simulink model "CF009A_GmOvrlStMgr"  (R2013b)
settings: Solver=FixedStepDiscrete  SolverMode=SingleTasking  StartTime=0.0  StopTime=1  FixedStep=0.002  RelTol=1e-3
values from neighbouring files (symbols this model uses):
  APASTACTV_CNT_U08 = DataDict.Constant    [CF009A_GmOvrlStMgr_DataDict.m]
  APASTCTRLAVL_CNT_U08 = DataDict.Constant    [CF009A_GmOvrlStMgr_DataDict.m]
  ARCHGLBPRM_2MILLISEC_SEC_F32 = DataDict.Constant    [CF009A_GmOvrlStMgr_DataDict.m]
  GmOvrlStMgrApaHwTqThd = DataDict.Calibration    [CF009A_GmOvrlStMgr_DataDict.m]
  GmOvrlStMgrApaHwTqTiThd = DataDict.Calibration    [CF009A_GmOvrlStMgr_DataDict.m]
  GmOvrlStMgrApaMfgEna = DataDict.Calibration    [CF009A_GmOvrlStMgr_DataDict.m]
  GmOvrlStMgrEscMfgEna = DataDict.Calibration    [CF009A_GmOvrlStMgr_DataDict.m]
  GmOvrlStMgrHaptcAmp = DataDict.Calibration    [CF009A_GmOvrlStMgr_DataDict.m]
  GmOvrlStMgrHaptcDurn = DataDict.Calibration    [CF009A_GmOvrlStMgr_DataDict.m]
  GmOvrlStMgrHaptcFrq = DataDict.Calibration    [CF009A_GmOvrlStMgr_DataDict.m]
  GmOvrlStMgrHaptcReactnTi = DataDict.Calibration    [CF009A_GmOvrlStMgr_DataDict.m]
  GmOvrlStMgrHaptcReqTiThd = DataDict.Calibration    [CF009A_GmOvrlStMgr_DataDict.m]
  GmOvrlStMgrHwAgTarLimr = DataDict.Calibration    [CF009A_GmOvrlStMgr_DataDict.m]
  GmOvrlStMgrLkaHwTqThd1 = DataDict.Calibration    [CF009A_GmOvrlStMgr_DataDict.m]
  GmOvrlStMgrLkaHwTqThd2 = DataDict.Calibration    [CF009A_GmOvrlStMgr_DataDict.m]
  GmOvrlStMgrLkaHwTqTiThd1 = DataDict.Calibration    [CF009A_GmOvrlStMgr_DataDict.m]
  GmOvrlStMgrLkaHwTqTiThd2 = DataDict.Calibration    [CF009A_GmOvrlStMgr_DataDict.m]
  GmOvrlStMgrLkaMfgEna = DataDict.Calibration    [CF009A_GmOvrlStMgr_DataDict.m]
  GmOvrlStMgrLoaMtgtnHaptcFbOffTi = DataDict.Calibration    [CF009A_GmOvrlStMgr_DataDict.m]
  GmOvrlStMgrLoaMtgtnHaptcFbOnTi = DataDict.Calibration    [CF009A_GmOvrlStMgr_DataDict.m]
  GmOvrlStMgrLoaMtgtnHaptcFbStrtOnTi = DataDict.Calibration    [CF009A_GmOvrlStMgr_DataDict.m]
  GmOvrlStMgrLoaMtgtnHaptcFbTqMax = DataDict.Calibration    [CF009A_GmOvrlStMgr_DataDict.m]
  GmOvrlStMgrLoaMtgtnHaptcFbTqMin = DataDict.Calibration    [CF009A_GmOvrlStMgr_DataDict.m]
  GmOvrlStMgrLoaMtgtnHaptcFbVehSpdMax = DataDict.Calibration    [CF009A_GmOvrlStMgr_DataDict.m]
  GmOvrlStMgrLoaMtgtnHaptcFbVehSpdMin = DataDict.Calibration    [CF009A_GmOvrlStMgr_DataDict.m]
  GmOvrlStMgrLoaMtgtnHaptcFrq = DataDict.Calibration    [CF009A_GmOvrlStMgr_DataDict.m]
  GmOvrlStMgrLoaMtgtnStrtHaptcAmp = DataDict.Calibration    [CF009A_GmOvrlStMgr_DataDict.m]
  GmOvrlStMgrLoaStIgnCntrThd = DataDict.Calibration    [CF009A_GmOvrlStMgr_DataDict.m]
  GmOvrlStMgrShiftLvrTiThd = DataDict.Calibration    [CF009A_GmOvrlStMgr_DataDict.m]
  GmOvrlStMgrStandStillThd = DataDict.Calibration    [CF009A_GmOvrlStMgr_DataDict.m]
  GmOvrlStMgrStandStillTiThd = DataDict.Calibration    [CF009A_GmOvrlStMgr_DataDict.m]
  HAPTCSTACTV_CNT_U08 = DataDict.Constant    [CF009A_GmOvrlStMgr_DataDict.m]
  HAPTCSTWAIT_CNT_U08 = DataDict.Constant    [CF009A_GmOvrlStMgr_DataDict.m]
  HWOSCNFRQMIN_HZ_F32 = DataDict.Constant    [CF009A_GmOvrlStMgr_DataDict.m]
  LKAFLTCNTRTHD_CNT_U08 = DataDict.Constant    [CF009A_GmOvrlStMgr_DataDict.m]
  LKAFLTTMRTHD_MILLISEC_U32 = DataDict.Constant    [CF009A_GmOvrlStMgr_DataDict.m]
  LKASTPRMNTFAILD_CNT_U08 = DataDict.Constant    [CF009A_GmOvrlStMgr_DataDict.m]
  MILLISECTO100MICROSECCNVN_CNT_U32 = DataDict.Constant    [CF009A_GmOvrlStMgr_DataDict.m]
  NODEBSTEP_CNT_U16 = DataDict.Constant    [CF009A_GmOvrlStMgr_DataDict.m]
undefined symbols (not defined in the file or in its folder): LoaSt1, NtcNr1, NtcSts1, NVM_RequestResultType, SysSt1
libraries: simulink x15, Fil x6, NxtrNvM x4, NxtrLim x4, NxtrAbslt x3, NxtrSign x2, FixdToFloat x1, FloatToFixd x1, LnrIntrpn x1
(part 2 of 8)

== stateflow chart CF009A_GmOvrlStMgr/GmOvrlStMgr/GmOvrlStMgrPer1/Chart ==
  state ESC [parallel]
    settings: executionOrder=1
    state Inactive
      entry:
      EscSt =ESCSTINACTV_CNT_U08 ;
    state Permanently_Failed
      entry:
      EscSt = ESCSTPRMNTFAILD_CNT_U08;
    state Active
      entry:
      EscSt = ESCSTACTV_CNT_U08;
    state Temporarily_Limited
      entry:
      EscSt = ESCSTTMPLIMD_CNT_U08;
    state Manufacturing_Disable
      entry:
      EscSt = ESCSTMFGDI_CNT_U08;
    (default) -> ESC.Inactive [order 2]
    ESC.Inactive -> ESC.Permanently_Failed [order 1] : [(EscFlt) || (LoaSt==LoaSt1.LOAST_SWBASDMTGTN)]
    ESC.Temporarily_Limited -> ESC.Inactive [order 2] : [~EscEna && (SysSt == SysSt1.SYSST_ENA)]
    ESC.Permanently_Failed -> ESC.Inactive : [((~EscEna) && (~EscFlt))&& ...
        | (LoaSt== LOASTNORM_CNT_U08)]
    ESC.Inactive -> ESC.Active [order 2] : [(EscEna) &&...
        | (VehSpdSecurMax <=GmOvrlStMgrEscVehSpdHiLim)]
    ESC.Active -> ESC.Inactive [order 2] : [(~EscEna)||...
        | (VehSpdSecurMax>GmOvrlStMgrEscVehSpdHiLim)]
    ESC.Active -> ESC.Permanently_Failed [order 1] : [EscFlt || (LoaSt==LoaSt1.LOAST_SWBASDMTGTN)]
    ESC.Temporarily_Limited -> ESC.Active [order 3] : [~EscLimdActv &&  (SysSt == SysSt1.SYSST_ENA)]
    ESC.Temporarily_Limited -> ESC.Permanently_Failed [order 1] : [(EscFlt ||...
        |  (LoaSt==LoaSt1.LOAST_SWBASDMTGTN))]
    ESC.Active -> ESC.Temporarily_Limited [order 3] : [(SysSt == SysSt1.SYSST_DI) || ...
        |  (EscLimdActv)]
    (default) -> ESC.Manufacturing_Disable [order 1] : [~EscMfgEna]
  state APA [parallel]
    settings: executionOrder=3
    state APANormal
      state TemporarilyInhibited
        entry:
        ApaSt = APASTTMPINHB_CNT_U08;
      state Available_for_Control
        entry:
        ApaSt = APASTCTRLAVL_CNT_U08;
        exit:
        HaptcSt = HAPTCSTINACTVNOTPLS_CNT_U08;
        state Not_Pulsing
          entry:
          HaptcSt = HAPTCSTINACTVNOTPLS_CNT_U08;
        state Pulsing
          state Pulse_Running
            entry:
            HaptcSt = HAPTCSTACTV_CNT_U08;
          state Waiting_After_Pulse
            entry:
            HaptcSt = HAPTCSTWAIT_CNT_U08;
          (default) -> Pulse_Running
          Pulse_Running -> Waiting_After_Pulse : [HaptcStTranActvToWaitFlg]
        state Ready_to_Pulse
          entry:
          HaptcSt = HAPTCSTINACTVRDYTOPLS_CNT_U08;
        state Pulse_Disabled
          entry:
          HaptcSt = HAPTCSTDI_CNT_U08;
        (default) -> Not_Pulsing [order 2]
        Pulsing -> Not_Pulsing : [(~VehStandStillTiExcdd) ||...
            |  (~ShiftLvrRvsTiExcdd) ||...
            |  (~ApaEna)]
        Not_Pulsing -> Ready_to_Pulse : [~HwHaptcEna]
        Ready_to_Pulse -> Not_Pulsing [order 2] : [HwHaptcEna]
        Ready_to_Pulse -> Pulsing [order 1] : [(VehStandStillTiExcdd) &&...
            |  (ShiftLvrRvsTiExcdd) &&...
            |  (ApaEna) &&...
            |  (HwHaptcEna)]
        (default) -> Pulse_Disabled [order 1] : [~GmOvrlStMgrApaHaptcEna]
      state Permanently_Failed
        entry:
        ApaSt =APASTPRMNTFAILD_CNT_U08 ;
      state Manufacturing_Disable
        entry:
        ApaSt = APASTMFGDI_CNT_U08;
      state Active
        entry:
        ApaSt =APASTACTV_CNT_U08;
      (default) -> TemporarilyInhibited [order 2]
      TemporarilyInhibited -> APA.APANormal.Permanently_Failed [order 1] : [(ApaNrcvrlFlt || ...
          | (LoaSt==LoaSt1.LOAST_SWBASDMTGTN))]
      APA.APANormal.Active -> TemporarilyInhibited [order 2] : [(SysSt == SysSt1.SYSST_DI) || ...
          |  (VehSpdSecurMax > GmOvrlStMgrApaVehSpdHiLim) ||...
          |  (ApaRcvrlFlt) ||...
          |  (HwHaptcEna) || ...
          |  (ApaIntv)]
      Available_for_Control -> TemporarilyInhibited [order 2] : [(SysSt == SysSt1.SYSST_DI) || ...
          |  (VehSpdSecurMax > GmOvrlStMgrApaVehSpdHiLim) ||...
          |  (ApaRcvrlFlt) ||...
          |  ((HwHaptcEna) && (HwHaptcEnaDurnExcdd))]
      TemporarilyInhibited -> Available_for_Control [order 2] : [(VehSpdSecurMax <= GmOvrlStMgrApaVehSpdHiLim) &&...
          |  (~ApaEna) &&...
          |  (~HwHaptcEna) &&...
          |  (~ApaRcvrlFlt)&&...
          | (SysSt == SysSt1.SYSST_ENA)]
      Available_for_Control -> APA.APANormal.Permanently_Failed [order 1] : [ApaNrcvrlFlt ||(LoaSt==LoaSt1.LOAST_SWBASDMTGTN)]
      APA.APANormal.Active -> APA.APANormal.Permanently_Failed [order 1] : [ApaNrcvrlFlt ||(LoaSt==LoaSt1.LOAST_SWBASDMTGTN)]
      Waiting_After_Pulse -> APA.APANormal.Active : [TranHaptcWaitToApaStActvFlg]
      Pulse_Disabled -> APA.APANormal.Active : [(VehStandStillTiExcdd) &&...
          |  (ShiftLvrRvsTiExcdd) &&...
          |  (ApaEna)]
      APA.APANormal.Active -> Available_for_Control [order 3] : [~ApaEna]
      (default) -> APA.APANormal.Manufacturing_Disable [order 1] : [~ApaMfgEna]
    (default) -> APANormal
  state LKA [parallel]
    settings: executionOrder=2
    state Inactive
      entry:
      LkaSt = LKASTINACTV_CNT_U08;
    state Temporarily_Limited
      entry:
      LkaSt = LKASTTMPLIMD_CNT_U08;
    state Active
      entry:
      LkaSt = LKASTACTV_CNT_U08;
    state Permanently_Failed
      entry:
      LkaSt = LKASTPRMNTFAILD_CNT_U08;
    state Manufacturing_Disable
      entry:
      LkaSt = LKASTMFGDI_CNT_U08;
    (default) -> LKA.Inactive [order 2]
    LKA.Temporarily_Limited -> LKA.Inactive [order 2] : [~LkaEna && (SysSt == SysSt1.SYSST_ENA)]
    LKA.Inactive -> LKA.Permanently_Failed [order 1] : [LkaPrmntFlt||(LoaSt==LoaSt1.LOAST_SWBASDMTGTN)]
    LKA.Inactive -> LKA.Temporarily_Limited [order 2] : [(SysSt == SysSt1.SYSST_DI) || ...
        |   ( (LkaEna) &&...
        |     ( (LkaFlt) ||...
        |       (LkaInhb) ||...
        |       (EscSt==ESCSTACTV_CNT_U08) ||...
        |       (EscSt==ESCSTTMPLIMD_CNT_U08)...
        |      )...
        |   )]
    LKA.Inactive -> LKA.Active [order 3] : [LkaEna &&...
        | (VehSpdSecurMin > GmOvrlStMgrLkaVehSpdLoLim) &&...
        | (VehSpdSecurMax < GmOvrlStMgrLkaVehSpdHiLim)]
    LKA.Active -> LKA.Inactive [order 2] : [(VehSpdSecurMin < GmOvrlStMgrLkaVehSpdLoLim) ||...
        |  (VehSpdSecurMax > GmOvrlStMgrLkaVehSpdHiLim) ||...
        |  (~LkaEna)]
    LKA.Active -> LKA.Permanently_Failed [order 1] : [LkaPrmntFlt|| (LoaSt==LoaSt1.LOAST_SWBASDMTGTN)]
    LKA.Active -> LKA.Temporarily_Limited [order 3] : [(SysSt == SysSt1.SYSST_DI) || ...
        |  ((LkaFlt) ||...
        |   (LkaInhb) ||...
        |   (LKAIntv) || ...
        |   (EscSt==ESCSTACTV_CNT_U08) || ...
        |   (EscSt==ESCSTTMPLIMD_CNT_U08)...
        |  ) ]
    LKA.Temporarily_Limited -> LKA.Permanently_Failed [order 1] : [(LkaPrmntFlt ||...
        |  (LoaSt==LoaSt1.LOAST_SWBASDMTGTN))]
    (default) -> LKA.Manufacturing_Disable [order 1] : [~LkaMfgEna]
  note: Nexteer Confidential -- Copyright 2013 Nexteer
  data: ApaSt output; VehSpdSecurMin input; VehSpdSecurMax input; ApaEna input; HwHaptcEna input; HwHaptcEnaDurnExcdd input; HaptcSt output uint8; VehStandStillTiExcdd input; ShiftLvrRvsTiExcdd input; ApaIntv input; ApaRcvrlFlt input; ApaNrcvrlFlt input; LkaSt output; LkaEna input; LkaFlt input; LkaInhb input; LkaPrmntFlt input; GmOvrlStMgrApaVehSpdHiLim parameter; GmOvrlStMgrLkaVehSpdHiLim parameter; GmOvrlStMgrLkaVehSpdLoLim parameter; GmOvrlStMgrApaHaptcEna parameter; EscSt output; EscEna input; EscFlt input; EscLimdActv input; ApaMfgEna input; LkaMfgEna input; EscMfgEna input; GmOvrlStMgrEscVehSpdHiLim parameter; LoaSt input uint8; APASTACTV_CNT_U08 parameter; APASTCTRLAVL_CNT_U08 parameter; APASTMFGDI_CNT_U08 parameter; APASTPRMNTFAILD_CNT_U08 parameter; APASTTMPINHB_CNT_U08 parameter; ESCSTACTV_CNT_U08 parameter; ESCSTINACTV_CNT_U08 parameter; ESCSTMFGDI_CNT_U08 parameter; ESCSTPRMNTFAILD_CNT_U08 parameter; ESCSTTMPLIMD_CNT_U08 parameter; HAPTCSTACTV_CNT_U08 parameter; HAPTCSTINACTVNOTPLS_CNT_U08 parameter; HAPTCSTWAIT_CNT_U08 parameter; LKASTACTV_CNT_U08 parameter; LKASTINACTV_CNT_U08 parameter; LKASTMFGDI_CNT_U08 parameter; LKASTPRMNTFAILD_CNT_U08 parameter; LKASTTMPLIMD_CNT_U08 parameter; LKAIntv input; HaptcStTranActvToWaitFlg input; TranHaptcWaitToApaStActvFlg input; HAPTCSTINACTVRDYTOPLS_CNT_U08 parameter; HAPTCSTDI_CNT_U08 parameter; SysSt input; LOASTNORM_CNT_U08 parameter

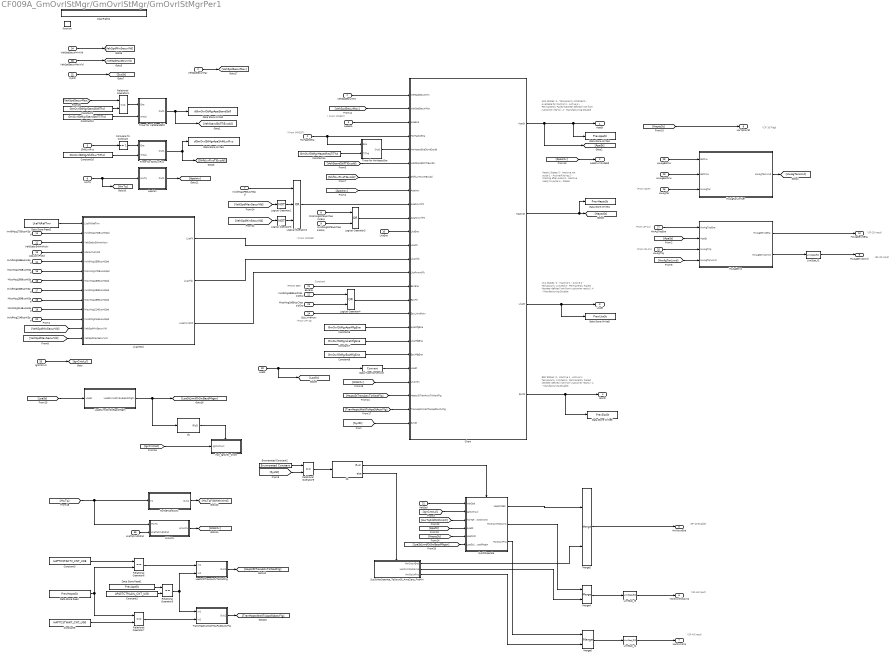
== system CF009A_GmOvrlStMgr/GmOvrlStMgr/GmOvrlStMgrPer1 ==
  note: ( From MM180)
  note: ( From MM337)
  note: ( From MM337)
  note: Constant
  note: (From SCIR)
  note: (From SF-21)
  note: (FROM SER)
  note: LKA States:
      |     0 - Inactive
      |     1 - Active
      |     2 - Temporarily Limited
      |     3 - Permanently Failed
      |
      | Nexteer defined (not from customer req'ts):
      |     4 - Manufacturing Disable
  note: APA States:
      |     0 - Temporarily Inhibited
      |     1 - Available for Control
      |     2 - Active
      |     3 - Permanently Failed
      |
      | Nexteer defined (not from customer req'ts):
      |     4 - Manufacturing Disable
  note: (SF-43 Enable)
  note: (SF-43 Input)
  note: (SF-43 Input)
  note: (CF-10 Flag)
  note: (From CF-10)
  note: ESC States:
      |     0 - Inactive
      |     1 - Active
      |     2 - Temporarily Limited
      |     3 - Permanently Failed
      |
      | Nexteer defined (not from customer req'ts):
      |     4 - Manufacturing Disable
  note: Haptic States
      |     0 - Inactive not pulse
      |     1 - Active/Pulsing
      |     2 - Waiting after pulse
      |     3 - Inactive ready to pulse
      |     4 - Diable
  note: (SF-20 Input)
  note: (SF-20 Input)
  note: (From SF-21)
  VehSpdSecurMin : Inport  RequirementInfo={} %GIDa_b0d3c35c_4503_4005_8ea2_9f2212553c6a
  VehSpdSecurMax : Inport  RequirementInfo={} %GIDa_e53e6896_dd80_42dc_965a_fcb79ee9124b  Port=2
  ApaEna : Inport  RequirementInfo={} %GIDa_8d1b5d03_8c5e_4c5e_91f3_bdd695e85069  Port=3
  HwHaptcEna : Inport  RequirementInfo={} %GIDa_06485b27_ab40_4ad3_bd14_ad4c2f62a393  Port=4
  ShiftLvrRvs : Inport  RequirementInfo={} %GIDa_dbbb7a9a_4381_48ec_960c_58daf9f19689  Port=5
  HwTq : Inport  RequirementInfo={} %GIDa_1ba3b84f_cb31_41a6_8598_2ca61152b6d2  Port=6
  InvldMsg1F5BusHiSpd : Inport  RequirementInfo={} %GIDa_f9b8db8c_5ec9_4279_8101_3b3cb8e96ee5  Port=7
  MissMsg337BusChassisExp : Inport  RequirementInfo={} %GIDa_2a54828a_623d_4a68_a97f_ee6c81b0f13e  Port=8
  InvldMsg337BusChassisExp : Inport  RequirementInfo={} %GIDa_a49582db_91ce_41e4_8ea7_fdb3beb7f641  Port=9
  LkaEna : Inport  RequirementInfo={} %GIDa_c67f821d_a534_4859_991f_be754908d78a  Port=10
  InvldMsg17DBusHiSpd : Inport  RequirementInfo={} %GIDa_c076c772_eeab_449c_b484_472e0cc8ed94  Port=11
  VehStabyEnhmtActv : Inport  RequirementInfo={} %GIDa_d5abf950_7af4_40d5_9676_0be52ecf66dc  Port=12
  AbsActvProtd : Inport  RequirementInfo={} %GIDa_04825455_bd19_4a90_9118_99efddee4468  Port=13
  InvldMsg1E9BusHiSpd : Inport  RequirementInfo={} %GIDa_ac4e6f02_8e0b_4fad_9ad8_288bf6f696c2  Port=14
  MissMsg17DBusHiSpd : Inport  RequirementInfo={} %GIDa_fcbc91b2_5e8e_4fde_b293_feb4eb68ea1d  Port=15
  MissMsg180BusHiSpd : Inport  RequirementInfo={} %GIDa_5a4e98da_8e0e_4ded_8f2b_0b345abaefca  Port=16
  InvldMsg180BusHiSpd : Inport  RequirementInfo={} %GIDa_c8d0ce3f_644b_4f0b_b33b_1e2f6d27c9df  Port=17
  MissMsg1E9BusHiSpd : Inport  RequirementInfo={} %GIDa_6ee56723_44b7_42b6_81ab_70915cbf1039  Port=18
  MissMsg214BusHiSpd : Inport  RequirementInfo={} %GIDa_9b7d257f_e0dc_4c9e_80ad_4a379171a5c2  Port=19
  InvldMsg214BusHiSpd : Inport  RequirementInfo={} %GIDa_ac526c57_18d5_4464_a148_218d3bfa9251  Port=20
  EscEna : Inport  RequirementInfo={} %GIDa_b7127805_3263_4184_831a_fc6c9b2cc01a  Port=21
  InvldMsg180BusChassisExp : Inport  RequirementInfo={} %GIDa_9ef29787_08e6_4663_a122_36a87bb12d59  Port=22
  MissMsg180BusChassisExp : Inport  RequirementInfo={} %GIDa_58661bb7_935e_4aa5_b2cb_a8077cff621a  Port=23
  EscLimdActv : Inport  RequirementInfo={} %GIDa_b1f90e60_6bab_4611_8ad9_e41738359040  Port=24
  HwAgTraj : Inport  RequirementInfo={} %GIDa_d5ec0ae6_f9e7_41b2_bf71_b480815ec2e8  Port=25
  HwAgTar : Inport  RequirementInfo={} %GIDa_6d588383_a210_4589_8f75_f9a00bf487c4  Port=26
  HwAgTrajEna : Inport  RequirementInfo={} %GIDa_30a153ec_8bbd_4ae8_86d5_91622ecf057d  Port=27
  HwAgEotCw : Inport  RequirementInfo={} %GIDa_a50a5d22_edbb_46ee_a5b7_bf143e2be1e6  Port=28
  HwAgEotCcw : Inport  RequirementInfo={} %GIDa_e08702f0_b186_40e1_9d5d_bab753fad415  Port=29
  LoaSt : Inport  RequirementInfo={} %GIDa_6f65a69f_1af1_4842_b860_3f517f73d3e8  Port=30  OutDataTypeStr=Enum: LoaSt1
  VehSpd : Inport  RequirementInfo={} %GIDa_198a1be4_59f5_4e8c_9975_df192cdf1251  Port=31
  SysSt : Inport  RequirementInfo={} %GIDa_5d1f0e27_a7b9_4b52_8773_b774a1daf0f1  Port=32
  IgnCntrLcl : Inport  RequirementInfo={} %GIDa_e0ba004e_4503_44da_8652_b13ad7bc9694  Port=33
  VehSpdSecurMinVld : Inport  RequirementInfo={} %GIDa_8aa24ca1_68b2_4a9c_89a4_0495831d4359  Port=34
  VehSpdSecurMaxVld : Inport  RequirementInfo={} %GIDa_dc311978_557e_4d2a_9a37_0f77a83cb914  Port=35
  "LkaTqCmdCdnd " : Inport  RequirementInfo={} %GIDa_6a679366_d481_4ed4_897f_c24ea9a03044  Port=36
  function : TriggerPort  TriggerType=function-call  PortDimensions=1
  ApaIntv : Subsystem
  Chart : Stateflow chart  RequirementInfo="{}  %GIDa_82f8cf8a_e966_40c9_996b_fc039507f794"  TreatAsAtomicUnit=on
  Compare To Constant : simulink/Logic and Bit Operations/Compare To Constant  relop===  const=1  OutDataTypeStr=boolean
  Constant1 : Constant  RequirementInfo={} %GIDa_7552fffd_837c_418f_a626_cb54a4ee4ecb  Value=GmOvrlStMgrStandStillThd
  Constant12 : Constant  RequirementInfo={} %GIDa_e0385d72_a04c_4c7f_8712_c1743adc4cad  Value=GmOvrlStMgrStandStillTiThd
  Constant14 : Constant  RequirementInfo={} %GIDa_4c34fc80_0be8_4916_b589_f77a913bde0d  Value=GmOvrlStMgrHaptcReqTiThd
  Constant16 : Constant  RequirementInfo={} %GIDa_414bbb4b_0344_45a0_913d_45c0053809cf  Value=GmOvrlStMgrShiftLvrTiThd
  Constant2 : Constant  Value=APASTCTRLAVL_CNT_U08
  Constant3 : Constant  Value=HAPTCSTACTV_CNT_U08
  Constant5 : Constant  Value=HAPTCSTWAIT_CNT_U08
  Constant6 : Constant  RequirementInfo={} %GIDa_6b44c89b_d793_4fde_b6dc_5afdec075d44  Value=GmOvrlStMgrApaMfgEna
  Constant7 : Constant  RequirementInfo={} %GIDa_f42bd636_c9a1_4d24_9506_dba1aeb30581  Value=GmOvrlStMgrLkaMfgEna
  Constant8 : Constant  RequirementInfo={} %GIDa_d43e135b_4699_428a_b5cf_b127f48922b5  Value=GmOvrlStMgrEscMfgEna
  CopyRight2 : Subsystem  Description=|  mask(Copyright Information){none=on}
      | Copyright info block.                                               
      |                                                                     
      | Place copyright information at the top of every subsystem in design.
      mask prompts: none "No parameters"
      mask help: Place copyright information at the top of every subsystem in design.
      mask Display:
      | NxtrConf = 'Nexteer Confidential';
      | 
      | sys = bdroot; %handle for the current model ("system")
      | first = get_param(sys,'Created');
      | first = first(end-3:end);  %year is last four digits
      | 
      | last = get_param(sys,'LastModifiedDate');
      | if isempty(last)
      |     last = datestr(now,'yyyy');
      | else
      |     last = last(end-3:end);
      | end
      | 
      | if strcmp(first,last)
      |     fprintf('%s -- Copyright %s Nexteer',NxtrConf,first)
      | else
      |     fprintf('%s -- %s%s- %s Nexteer',NxtrConf,char(169),first,last)
      | end
  Data Store Read : DataStoreRead  DataStoreName=PrevHaptcSt
  Data Store Read1 : DataStoreRead  DataStoreName=PrevApaSt
  Data Store Read2 : DataStoreRead  DataStoreName=LkaFltRefTmr
  Data Store Write1 : DataStoreWrite  DataStoreName=dGmOvrlStMgrApaShiftLvrRvs
  Data Store Write2 : DataStoreWrite  DataStoreName=dGmOvrlStMgrApaStandStill
  Data Store Write3 : DataStoreWrite  DataStoreName=PrevApaSt
  Data Store Write4 : DataStoreWrite  DataStoreName=PrevHaptcSt
  Data Store Write5 : DataStoreWrite  DataStoreName=PrevLkaSt
  Data Store Write6 : DataStoreWrite  DataStoreName=PrevEscSt
  Data Type Conversion : DataTypeConversion
  Enumerated Constant2 : simulink/Sources/Enumerated Constant  OutDataTypeStr=Enum: SysSt1  Value=SysSt1.SYSST_ENA  SampleTime=inf
  HaptcStTransActvToWaitFlg : Subsystem
  HwAgServo : Subsystem  RequirementInfo={} %GIDa_aaea10c3_5552_4f84_b64c_db5f293fc08c
  HwAgTarLimiter : Subsystem  RequirementInfo={} %GIDa_1c9b0e23_9620_4264_8618_d0192b732e95
  HwTqFildIntlChk : Subsystem
  If1 : If  IfExpression=u1  ShowElse=off
  If4 : If  IfExpression=u1
  Inct_IgnCntr_Once : Subsystem
  LKAIntv : Subsystem
  LimStat_f1 : NxtrLim/LimStat_f32  LoLim=HWAGSERVOCMDMIN_HWDEG_F32  HiLim=HWAGSERVOCMDMAX_HWDEG_F32
      settings: AttributesFormatString=|
      | Low Limit: %<LoLim>
      | High Limit:%<HiLim>
  LimStat_f3 : NxtrLim/LimStat_f32  LoLim=HWOSCNMOTAMPMIN_MOTNWTMTR_F32  HiLim=HWOSCNMOTAMPMAX_MOTNWTMTR_F32
      settings: AttributesFormatString=|
      | Low Limit: %<LoLim>
      | High Limit:%<HiLim>
  LimStat_f4 : NxtrLim/LimStat_f32  LoLim=HWOSCNFRQMIN_HZ_F32  HiLim=HWOSCNFRQMAX_HZ_F32
      settings: AttributesFormatString=|
      | Low Limit: %<LoLim>
      | High Limit:%<HiLim>
  LkaCheck : Subsystem
  LoaStLimdOrSwBasdMtgtn : Subsystem
  Logical Operator1 : Logic  Operator=NOT  AllPortsSameDT=off  OutDataTypeStr=boolean
  Logical Operator2 : Logic  Operator=OR  Inputs=3  AllPortsSameDT=off  OutDataTypeStr=boolean
  Logical Operator3 : Logic  Operator=OR  AllPortsSameDT=off  OutDataTypeStr=boolean
  Logical Operator4 : Logic  Operator=OR  AllPortsSameDT=off  OutDataTypeStr=boolean
  Logical Operator5 : Logic  Operator=NOT  AllPortsSameDT=off  OutDataTypeStr=boolean
  Merge4 : Merge
  Merge5 : Merge
  Merge6 : Merge
  Relational Operator3 : RelationalOperator  Operator=<=  OutDataTypeStr=boolean
  Relational Operator{5..7,9} (4 alike) : RelationalOperator  Operator===  OutDataTypeStr=boolean
  SysStNotOperate_TqOscnDi_AmpZero_FrqMin : Subsystem
  SysStOperate : Subsystem  TreatAsAtomicUnit=on
  Timer for HwHaptcEna : Subsystem
  Timer for ShiftLvrRvs : Subsystem
  Timer for VehStandStill : Subsystem
  TransHaptcsWaitToAPAStActvFlg : Subsystem
  ApaSt : Outport  RequirementInfo={} %GIDa_75635ebd_fcf5_4cad_9536_b406ee611602
  ApaDrvrIntvDetd : Outport  RequirementInfo={} %GIDa_1797abc3_35b6_41e8_9538_2064f4102f87  Port=2
  LkaSt : Outport  RequirementInfo={} %GIDa_686c82ef_a42d_4546_a1da_a62cef7fe954  Port=3
  EscSt : Outport  RequirementInfo={} %GIDa_ad72c3fe_3139_49da_a979_17fad9a56d26  Port=4
  HwOscnEna : Outport  RequirementInfo={} %GIDa_d848a758_683b_4a9d_a345_2c9338079af2  Port=5
  HwOscnMotAmp : Outport  RequirementInfo={} %GIDa_159c2416_70a4_4698_a3a2_bfc8caad832f  Port=6
  HwOscnFrq : Outport  RequirementInfo={} %GIDa_bf0dab85_578c_4235_861d_cc8928b85320  Port=7
  HwTqOscSt : Outport  RequirementInfo={} %GIDa_f57d728d_5e71_4f6a_bae2_eb0c6758b489  Port=8
  HwAgServoCmd : Outport  RequirementInfo={} %GIDa_a0e1e034_04e0_4255_bc05_d7a545e9e511  Port=9
  HwAgServoEna : Outport  RequirementInfo={} %GIDa_e4571625_3f2f_4611_bb8a_43a258de8b52  Port=10
  wires:
  EscLimdActv/1 -> Chart/17(EscLimdActv)
  HwAgTraj/1 -> HwAgServo/3(HwAgTraj)
  HwAgTar/1 -> HwAgTarLimiter/3(HwAgTar)
  Chart/1(ApaSt) -> ApaSt/1, Data Store Write3/1, [ApaSt]
  EscEna/1 -> Chart/15(EscEna)
  HwAgEotCcw/1 -> HwAgTarLimiter/2(EotCcw)
  HwHaptcEna/1 -> Timer for HwHaptcEna/1(Ena), Chart/4(HwHaptcEna)
  [HaptcSt] -> HwTqOscSt/1
  Logical Operator4/1 -> Chart/16(EscFlt)
  HwAgTarLimiter/1(HwAgTarLimd) -> [HwAgTarLimd]
  ApaEna/1 -> Chart/3(ApaEna)
  Chart/4(EscSt) -> EscSt/1, Data Store Write6/1
  Chart/3(LkaSt) -> LkaSt/1, Data Store Write5/1
  HwAgServo/1(HwAgServoEna) -> HwAgServoEna/1
  Logical Operator2/1 -> Chart/9(ApaRcvrlFlt)
  HwAgTrajEna/1 -> HwAgServo/1(HwAgTrajEna)
  HwAgEotCw/1 -> HwAgTarLimiter/1(EotCw)
  Timer for HwHaptcEna/1(Out1) -> Chart/5(HwHaptcEnaDurnExcdd)
  Chart/2(HaptcSt) -> Data Store Write4/1, [HaptcSt]
  HwAgServo/2(HwAgServoCmd) -> LimStat_f1/1
  [ApaIntv] -> ApaDrvrIntvDetd/1
  [HwAgTarLimd] -> HwAgServo/4(HwAgTarLimd)
  Logical Operator3/1 -> Chart/10(ApaNrcvrlFlt)
  LoaSt/1 -> Data Type Conversion/1, [LoaSt]
  Constant14/1 -> Timer for HwHaptcEna/2(TiThd)
  ApaIntv/1(Out1) -> [ApaIntv]
  [ApaIntv] -> Chart/8(ApaIntv)
  Timer for VehStandStill/1(Out1) -> [VehStandStillTiExcdd], Data Store Write2/1
  [VehStandStillTiExcdd] -> Chart/6(VehStandStillTiExcdd)
  Timer for ShiftLvrRvs/1(Out1) -> [ShiftLvrRvsTiExcdd], Data Store Write1/1
  ShiftLvrRvs/1 -> Compare To Constant/1
  [ShiftLvrRvsTiExcdd] -> Chart/7(ShiftLvrRvsTiExcdd)
  [VehSpdSecurMax] -> Chart/2(VehSpdSecurMax)
  [ApaSt] -> HwAgServo/2(ApaSt)
  LkaEna/1 -> Chart/11(LkaEna)
  Constant12/1 -> Timer for VehStandStill/2(TiThd)
  Constant1/1 -> Relational Operator3/2
  Relational Operator3/1 -> Timer for VehStandStill/1(Ena)
  Constant16/1 -> Timer for ShiftLvrRvs/2(TiThd)
  Compare To Constant/1 -> Timer for ShiftLvrRvs/1(Ena)
  InvldMsg1F5BusHiSpd/1 -> Logical Operator2/1
  InvldMsg337BusChassisExp/1 -> Logical Operator3/2
  MissMsg337BusChassisExp/1 -> Logical Operator3/1
  InvldMsg180BusChassisExp/1 -> Logical Operator4/1
  MissMsg180BusChassisExp/1 -> Logical Operator4/2
  HwTq/1 -> [HwTq], ApaIntv/1(HwTq)
  Data Type Conversion/1 -> Chart/21(LoaSt)
  LimStat_f3/1 -> HwOscnMotAmp/1
  LimStat_f4/1 -> HwOscnFrq/1
  HwTqFildIntlChk/1(Out1) -> [HwTqFildWithinIntl]
  LKAIntv/1(LKAIntv) -> [LKAIntv]
  [LKAIntv] -> Chart/22(LKAIntv)
  LimStat_f1/1 -> HwAgServoCmd/1
  HaptcStTransActvToWaitFlg/1(Out1) -> [HaptcStTranActvToWaitFlg]
  TransHaptcsWaitToAPAStActvFlg/1(Out1) -> [TranHaptcWaitToApaStActvFlg]
  [HaptcStTranActvToWaitFlg] -> Chart/23(HaptcStTranActvToWaitFlg)
  [TranHaptcWaitToApaStActvFlg] -> Chart/24(TranHaptcWaitToApaStActvFlg)
  Data Store Read1/1 -> Relational Operator5/1
  Constant2/1 -> Relational Operator5/2
  Relational Operator5/1 -> TransHaptcsWaitToAPAStActvFlg/1(In1), HaptcStTransActvToWaitFlg/2(In2)
  Constant3/1 -> Relational Operator6/1
  Data Store Read/1 -> Relational Operator7/1, Relational Operator6/2
  Constant5/1 -> Relational Operator7/2
  Relational Operator7/1 -> TransHaptcsWaitToAPAStActvFlg/2(In2)
  Relational Operator6/1 -> HaptcStTransActvToWaitFlg/1(In1)
  If4/1 -> SysStOperate/Action
  If4/2 -> SysStNotOperate_TqOscnDi_AmpZero_FrqMin/Action
  Relational Operator9/1 -> If4/1
  Enumerated Constant2/1 -> Relational Operator9/1
  SysStOperate/2(HwOscnMotAmp) -> Merge4/1
  SysStOperate/1(HaptcFbEn) -> Merge5/1
  SysStOperate/3(HwOscnFrq) -> Merge6/1
  SysStNotOperate_TqOscnDi_AmpZero_FrqMin/1(HwOscnEna) -> Merge5/2
  SysStNotOperate_TqOscnDi_AmpZero_FrqMin/3(HwOscnFrq) -> Merge6/2
  SysStNotOperate_TqOscnDi_AmpZero_FrqMin/2(HwOscnMotAmp) -> Merge4/2
  Merge5/1 -> HwOscnEna/1
  Merge6/1 -> LimStat_f4/1
  Merge4/1 -> LimStat_f3/1
  VehSpd/1 -> SysStOperate/1(VehSpd)
  [ApaSt] -> SysStOperate/4(ApaSt)
  [HaptcSt] -> SysStOperate/5(HaptcSt)
  [HwTqFildWithinIntl] -> SysStOperate/3(HwTqFildWithinIntl)
  Constant6/1 -> Chart/18(ApaMfgEna)
  Constant7/1 -> Chart/19(LkaMfgEna)
  Constant8/1 -> Chart/20(EscMfgEna)
  [IgnCntrLcl] -> SysStOperate/2(IgnCntrLcl)
  If1/1 -> Inct_IgnCntr_Once/Action
  LoaStLimdOrSwBasdMtgtn/1(LoaStLimdOrSwBasdMtgtn) -> [LoaStLimdOrSwBasdMtgtn], If1/1
  [IgnCntrLcl] -> Inct_IgnCntr_Once/1(IgnCntrLcl)
  [LoaSt] -> LoaStLimdOrSwBasdMtgtn/1(LoaSt)
  IgnCntrLcl/1 -> [IgnCntrLcl]
  [LoaStLimdOrSwBasdMtgtn] -> SysStOperate/6(LoaStLimdOrSwBasdMtgtn)
  [VehSpdSecurMax] -> Relational Operator3/1
  VehSpdSecurMin/1 -> Chart/1(VehSpdSecurMin)
  [VehSpdMaxSecurVld] -> Logical Operator1/1
  [VehSpdMinSecurVld] -> Logical Operator5/1
  LkaCheck/1(LkaFlt) -> Chart/12(LkaFlt)
  InvldMsg17DBusHiSpd/1 -> LkaCheck/2(InvldMsg17DBusHiSpd)
  VehStabyEnhmtActv/1 -> LkaCheck/3(VehStabyEnhmtActv)
  AbsActvProtd/1 -> LkaCheck/4(AbsActvProtd)
  InvldMsg1E9BusHiSpd/1 -> LkaCheck/5(InvldMsg1E9BusHiSpd)
  MissMsg17DBusHiSpd/1 -> LkaCheck/6(MissMsg17DBusHiSpd)
  MissMsg180BusHiSpd/1 -> LkaCheck/7(MissMsg180BusHiSpd)
  InvldMsg180BusHiSpd/1 -> LkaCheck/8(InvldMsg180BusHiSpd)
  MissMsg1E9BusHiSpd/1 -> LkaCheck/9(MissMsg1E9BusHiSpd)
  MissMsg214BusHiSpd/1 -> LkaCheck/10(MissMsg214BusHiSpd)
  InvldMsg214BusHiSpd/1 -> LkaCheck/11(InvldMsg214BusHiSpd)
  LkaCheck/2(LkaInhb) -> Chart/13(LkaInhb)
  LkaCheck/3(LkaPrmntFlt) -> Chart/14(LkaPrmntFlt)
  [VehSpdMaxSecurVld] -> LkaCheck/13(VehSpdMaxSecurVld)
  [VehSpdMinSecurVld] -> LkaCheck/12(VehSpdMinSecurVld)
  SysSt/1 -> [SysSt]
  [SysSt] -> Relational Operator9/2
  [SysSt] -> Chart/25(SysSt)
  VehSpdSecurMinVld/1 -> [VehSpdMinSecurVld]
  VehSpdSecurMaxVld/1 -> [VehSpdMaxSecurVld]
  Logical Operator1/1 -> Logical Operator2/2
  Logical Operator5/1 -> Logical Operator2/3
  VehSpdSecurMax/1 -> [VehSpdSecurMax]
  Data Store Read2/1 -> LkaCheck/1(LkaFltRefTmr)
  [HwTq] -> LKAIntv/1(HwTq), HwTqFildIntlChk/1(In1)
  "LkaTqCmdCdnd "/1 -> LKAIntv/2(LkaTqCmdCdnd)

== system CF009A_GmOvrlStMgr/GmOvrlStMgr/SetGmLoaIgnCntr ==
  GmLoaIgnCntr : Inport  RequirementInfo={} %GIDa_f6a28945_b2be_4817_8103_f6fab52ae2d6
  function : TriggerPort  TriggerType=function-call
  Constant1 : Constant  Value=true  OutDataTypeStr=boolean
      settings: AttributesFormatString=%<OutDataTypeStr>
  CopyRight2 : Subsystem  Description=|  mask(Copyright Information){none=on}
      | Copyright info block.                                               
      |                                                                     
      | Place copyright information at the top of every subsystem in design.
      mask prompts: none "No parameters"
      mask help: Place copyright information at the top of every subsystem in design.
      mask Display:
      | NxtrConf = 'Nexteer Confidential';
      | 
      | sys = bdroot; %handle for the current model ("system")
      | first = get_param(sys,'Created');
      | if(isempty(first))
      |     first = datestr(now,'yyyy');
      | else
      |     first = first(end-3:end);  %year is last four digits
      | end
      | 
      | last = get_param(sys,'LastModifiedDate');
      | if isempty(last)
      |     last = datestr(now,'yyyy');
      | else
      |     last = last(end-3:end);
      | end
      | 
      | if strcmp(first,last)
      |     fprintf('%s -- Copyright %s Nexteer',NxtrConf,first)
      | else
      |     fprintf('%s -- %s%s- %s Nexteer',NxtrConf,char(169),first,last)
      | end
  Data Store Write8 : DataStoreWrite  DataStoreName=GmLoaIgnCntr
  GmLoaIgnCntr_Set Ram Block Status : NxtrNvM/Set Ram Block Status  FuncName=Set Ram Block Status  NvMBlockName=GmLoaIgnCntr  VoidFuncRtn=on  BlockChanged_DSN=NvMSRBS_BlockChanged  Return_DSN=NvMSRBS_Return1
      settings: AttributesFormatString=%<FuncName>
  wires:
  GmLoaIgnCntr/1 -> Data Store Write8/1
  Constant1/1 -> GmLoaIgnCntr_Set Ram Block Status/1

== system CF009A_GmOvrlStMgr/call_GetGmLoaIgnCntr/CopyRight1 ==

== system CF009A_GmOvrlStMgr/call_GmOvrlStMgrInit1/CopyRight2 ==

== system CF009A_GmOvrlStMgr/call_GmOvrlStMgrPer1/CopyRight2 ==

== system CF009A_GmOvrlStMgr/call_SetGmLoaIgnCntr/CopyRight1 ==

== system CF009A_GmOvrlStMgr/GmOvrlStMgr/GetGmLoaIgnCntr/CopyRight2 ==

== system CF009A_GmOvrlStMgr/GmOvrlStMgr/GmOvrlStMgrInit1/CopyRight2 ==

== system CF009A_GmOvrlStMgr/GmOvrlStMgr/GmOvrlStMgrInit1/GetRefTmr100MicroSec32bit ==
  note: Created Aug 18, 2015
      | Modified Oct 21, 2015
      | Modified Oct 30, 2015
      | Kevin Derry
  note: GetRefTmr100MicroSec32bit
  note: Wrap-to-zero
  note: counts
  note: microseconds
  note: seconds
  note: 1 count = 100 uSec
  CopyRight2 : Subsystem  Description=|  mask(Copyright Information){none=on}
      | Copyright info block.                                               
      |                                                                     
      | Place copyright information at the top of every subsystem in design.
      mask prompts: none "No parameters"
      mask help: Place copyright information at the top of every subsystem in design.
      mask Display:
      | NxtrConf = 'Nexteer Confidential';
      | 
      | sys = bdroot; %handle for the current model ("system")
      | first = get_param(sys,'Created');
      | if(isempty(first))
      |     first = datestr(now,'yyyy');
      | else
      |     first = first(end-3:end);  %year is last four digits
      | end
      | 
      | last = get_param(sys,'LastModifiedDate');
      | if isempty(last)
      |     last = datestr(now,'yyyy');
      | else
      |     last = last(end-3:end);
      | end
      | 
      | if strcmp(first,last)
      |     fprintf('%s -- Copyright %s Nexteer',NxtrConf,first)
      | else
      |     fprintf('%s -- %s%s- %s Nexteer',NxtrConf,char(169),first,last)
      | end
  Count per uSec : Constant  Value=0.01
  Data Store Read1 : DataStoreRead  DataStoreName=SimnTi
  Data Type Conversion1 : DataTypeConversion  OutDataTypeStr=uint32
  Divide1 : Product  Inputs=**
  Divide2 : Product  Inputs=*/
  Max Counts : Constant  Value=2^32-1
  Product1 : Product
  Product2 : Product
  Rounding : Rounding
  Subtract1 : Sum  Inputs=+-
  uSec per Sec : Constant  Value=1000000
  RefTmr : Outport
  wires:
  Data Store Read1/1 -> Product1/1
  Data Type Conversion1/1 -> RefTmr/1
  uSec per Sec/1 -> Product1/2
  Count per uSec/1 -> Divide1/2
  Product1/1 -> Divide1/1
  Divide1/1 -> Subtract1/1, Divide2/1
  Max Counts/1 -> Product2/2, Divide2/2
  Divide2/1 -> Rounding/1
  Rounding/1 -> Product2/1
  Subtract1/1 -> Data Type Conversion1/1
  Product2/1 -> Subtract1/2

== system CF009A_GmOvrlStMgr/GmOvrlStMgr/GmOvrlStMgrInit1/NTC_Fault1_Set_Faild ==
  NtcNr : Inport
  NtcStInfo : Inport  Port=2
  NtcSts : Inport  Port=3
  DebStep : Inport  Port=4
  CallDiagMgr : ActionPort  ActionType=then
  SetNtcSts : Subsystem  RequirementInfo={} %GIDa_d459548b_e0d4_4661_8326_6b6064fa956f  TreatAsAtomicUnit=on
      settings: RTWSystemCode=Inline
  wires:
  NtcStInfo/1 -> SetNtcSts/2(NtcStInfo)
  DebStep/1 -> SetNtcSts/4(DebStep)
  NtcSts/1 -> SetNtcSts/3(NtcSts)
  NtcNr/1 -> SetNtcSts/1(NtcNr)  "NtcNr"

== system CF009A_GmOvrlStMgr/GmOvrlStMgr/GmOvrlStMgrInit1/NTC_Fault1_Set_Passd ==
  NtcNr : Inport
  NtcStInfo : Inport  Port=2
  NtcSts : Inport  Port=3
  DebStep : Inport  Port=4
  CallDiagMgr : ActionPort  ActionType=else
  SetNtcSts : Subsystem  RequirementInfo={} %GIDa_e624de36_990e_40b1_800e_f81e88e68b40  TreatAsAtomicUnit=on
      settings: RTWSystemCode=Inline
  wires:
  NtcNr/1 -> SetNtcSts/1(NtcNr)  "NtcNr"
  NtcSts/1 -> SetNtcSts/3(NtcSts)
  DebStep/1 -> SetNtcSts/4(DebStep)
  NtcStInfo/1 -> SetNtcSts/2(NtcStInfo)

== system CF009A_GmOvrlStMgr/GmOvrlStMgr/GmOvrlStMgrInit1/NVM_NOK ==
  note: In the event of NVM failure
      | zero out the shadow ram image
  Action Port : ActionPort  ActionType=then
  Constant1 : Constant  Value=0  OutDataTypeStr=uint16
      settings: AttributesFormatString=%<OutDataTypeStr>
  CopyRight2 : Subsystem  Description=|  mask(Copyright Information){none=on}
      | Copyright info block.                                               
      |                                                                     
      | Place copyright information at the top of every subsystem in design.
      mask prompts: none "No parameters"
      mask help: Place copyright information at the top of every subsystem in design.
      mask Display:
      | NxtrConf = 'Nexteer Confidential';
      | 
      | sys = bdroot; %handle for the current model ("system")
      | first = get_param(sys,'Created');
      | if(isempty(first))
      |     first = datestr(now,'yyyy');
      | else
      |     first = first(end-3:end);  %year is last four digits
      | end
      | 
      | last = get_param(sys,'LastModifiedDate');
      | if isempty(last)
      |     last = datestr(now,'yyyy');
      | else
      |     last = last(end-3:end);
      | end
      | 
      | if strcmp(first,last)
      |     fprintf('%s -- Copyright %s Nexteer',NxtrConf,first)
      | else
      |     fprintf('%s -- %s%s- %s Nexteer',NxtrConf,char(169),first,last)
      | end
  Data Store Write8 : DataStoreWrite  DataStoreName=GmLoaIgnCntr
  wires:
  Constant1/1 -> Data Store Write8/1

== system CF009A_GmOvrlStMgr/GmOvrlStMgr/GmOvrlStMgrInit1/NVM_Ok ==
  Action Port : ActionPort  ActionType=else
  Constant1 : Constant  Value=0  OutDataTypeStr=Inherit: Inherit via back propagation
  CopyRight2 : Subsystem  Description=|  mask(Copyright Information){none=on}
      | Copyright info block.                                               
      |                                                                     
      | Place copyright information at the top of every subsystem in design.
      mask prompts: none "No parameters"
      mask help: Place copyright information at the top of every subsystem in design.
      mask Display:
      | NxtrConf = 'Nexteer Confidential';
      | 
      | sys = bdroot; %handle for the current model ("system")
      | first = get_param(sys,'Created');
      | if(isempty(first))
      |     first = datestr(now,'yyyy');
      | else
      |     first = first(end-3:end);  %year is last four digits
      | end
      | 
      | last = get_param(sys,'LastModifiedDate');
      | if isempty(last)
      |     last = datestr(now,'yyyy');
      | else
      |     last = last(end-3:end);
      | end
      | 
      | if strcmp(first,last)
      |     fprintf('%s -- Copyright %s Nexteer',NxtrConf,first)
      | else
      |     fprintf('%s -- %s%s- %s Nexteer',NxtrConf,char(169),first,last)
      | end
  Terminator : Terminator
  wires:
  Constant1/1 -> Terminator/1

== system CF009A_GmOvrlStMgr/GmOvrlStMgr/GmOvrlStMgrInit1/Saturate ==
  In1 : Inport
  Action Port : ActionPort  ActionType=else
  Out1 : Outport
  wires:
  In1/1 -> Out1/1

== system CF009A_GmOvrlStMgr/GmOvrlStMgr/GmOvrlStMgrInit1/StepDown ==
  Acc : Inport
  Action Port : ActionPort  ActionType=then
  Constant1 : Constant  OutDataTypeStr=Inherit: Inherit via back propagation
  Constant8 : Constant  Value=true  OutDataTypeStr=boolean
      settings: AttributesFormatString=%<OutDataTypeStr>
  GmLoaIgnCntr_Set Ram Block Status : NxtrNvM/Set Ram Block Status  FuncName=Set Ram Block Status  NvMBlockName=GmLoaIgnCntr  VoidFuncRtn=on  BlockChanged_DSN=NvMSRBS_BlockChanged  Return_DSN=NvMSRBS_Return2
      settings: AttributesFormatString=%<FuncName>
  subtract : Sum  Inputs=+-
  NewAccum : Outport
  wires:
  subtract/1 -> NewAccum/1
  Constant1/1 -> subtract/2
  Acc/1 -> subtract/1
  Constant8/1 -> GmLoaIgnCntr_Set Ram Block Status/1

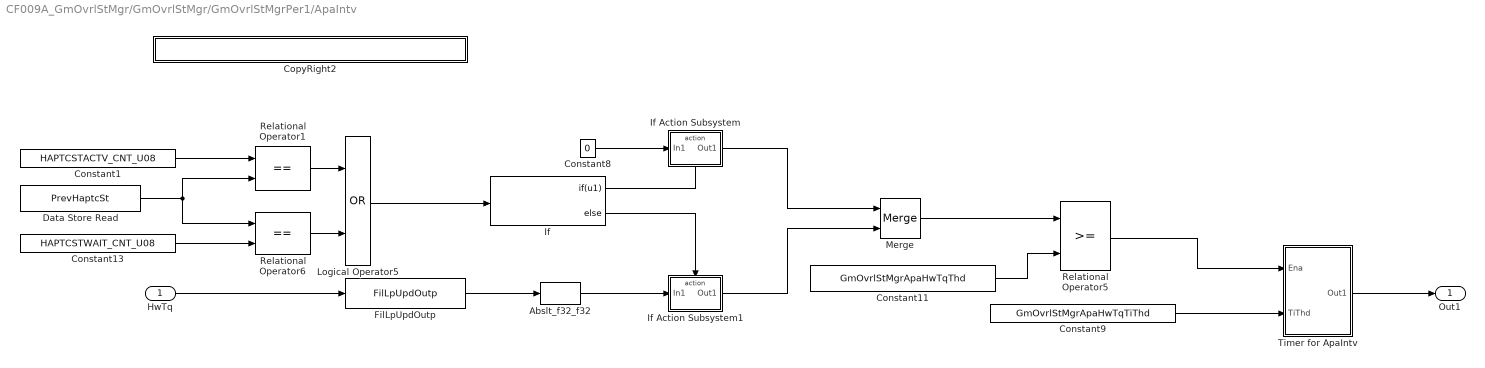
== system CF009A_GmOvrlStMgr/GmOvrlStMgr/GmOvrlStMgrPer1/ApaIntv ==
  HwTq : Inport
  Abslt_f32_f32 : NxtrAbslt/Abslt_f32_f32  SFunctionSpec=single y1 = Abslt_f32_f32(single u1)
      settings: AttributesFormatString=%<Name>
  Constant1 : Constant  Value=HAPTCSTACTV_CNT_U08  OutDataTypeStr=uint16
  Constant11 : Constant  RequirementInfo={} %GIDa_ec52fe9d_5e44_40e3_866f_d0086c13c635  Value=GmOvrlStMgrApaHwTqThd
  Constant13 : Constant  Value=HAPTCSTWAIT_CNT_U08  OutDataTypeStr=uint16
  Constant8 : Constant  Value=0  OutDataTypeStr=single
  Constant9 : Constant  RequirementInfo={} %GIDa_5c7ed4f2_0f89_4005_946e_0cb6eaa566b5  Value=GmOvrlStMgrApaHwTqTiThd
  CopyRight2 : Subsystem  Description=|  mask(Copyright Information){none=on}
      | Copyright info block.                                               
      |                                                                     
      | Place copyright information at the top of every subsystem in design.
      mask prompts: none "No parameters"
      mask help: Place copyright information at the top of every subsystem in design.
      mask Display:
      | NxtrConf = 'Nexteer Confidential';
      | 
      | sys = bdroot; %handle for the current model ("system")
      | first = get_param(sys,'Created');
      | first = first(end-3:end);  %year is last four digits
      | 
      | last = get_param(sys,'LastModifiedDate');
      | if isempty(last)
      |     last = datestr(now,'yyyy');
      | else
      |     last = last(end-3:end);
      | end
      | 
      | if strcmp(first,last)
      |     fprintf('%s -- Copyright %s Nexteer',NxtrConf,first)
      | else
      |     fprintf('%s -- %s%s- %s Nexteer',NxtrConf,char(169),first,last)
      | end
  Data Store Read : DataStoreRead  DataStoreName=PrevHaptcSt
  FilLpUpdOutp : Fil/FilLpUpdOutp  StVar=HwTqLpFil
      settings: AttributesFormatString=StVar: %<StVar>
  If : If  IfExpression=u1
  If Action Subsystem : Subsystem  TreatAsAtomicUnit=on
  If Action Subsystem1 : Subsystem  TreatAsAtomicUnit=on
  Logical Operator5 : Logic  Operator=OR  AllPortsSameDT=off  OutDataTypeStr=boolean
  Merge : Merge
  Relational Operator1 : RelationalOperator  Operator===  OutDataTypeStr=boolean
  Relational Operator5 : RelationalOperator  OutDataTypeStr=boolean
  Relational Operator6 : RelationalOperator  Operator===  OutDataTypeStr=boolean
  Timer for ApaIntv : Subsystem
  Out1 : Outport
  wires:
  Data Store Read/1 -> Relational Operator6/1, Relational Operator1/2
  If/1 -> If Action Subsystem/Action
  If/2 -> If Action Subsystem1/Action
  HwTq/1 -> FilLpUpdOutp/1
  If Action Subsystem/1(Out1) -> Merge/1
  If Action Subsystem1/1(Out1) -> Merge/2
  Constant8/1 -> If Action Subsystem/1(In1)
  Timer for ApaIntv/1(Out1) -> Out1/1
  FilLpUpdOutp/1 -> Abslt_f32_f32/1
  Constant13/1 -> Relational Operator6/2
  Relational Operator6/1 -> Logical Operator5/2
  Abslt_f32_f32/1 -> If Action Subsystem1/1(In1)
  Constant9/1 -> Timer for ApaIntv/2(TiThd)
  Merge/1 -> Relational Operator5/1
  Constant11/1 -> Relational Operator5/2
  Relational Operator5/1 -> Timer for ApaIntv/1(Ena)
  Constant1/1 -> Relational Operator1/1
  Relational Operator1/1 -> Logical Operator5/1
  Logical Operator5/1 -> If/1

== system CF009A_GmOvrlStMgr/GmOvrlStMgr/GmOvrlStMgrPer1/CopyRight2 ==

== system CF009A_GmOvrlStMgr/GmOvrlStMgr/GmOvrlStMgrPer1/HaptcStTransActvToWaitFlg ==
  In1 : Inport
  In2 : Inport  Port=2
  CopyRight2 : Subsystem  Description=|  mask(Copyright Information){none=on}
      | Copyright info block.                                               
      |                                                                     
      | Place copyright information at the top of every subsystem in design.
      mask prompts: none "No parameters"
      mask help: Place copyright information at the top of every subsystem in design.
      mask Display:
      | NxtrConf = 'Nexteer Confidential';
      | 
      | sys = bdroot; %handle for the current model ("system")
      | first = get_param(sys,'Created');
      | first = first(end-3:end);  %year is last four digits
      | 
      | last = get_param(sys,'LastModifiedDate');
      | if isempty(last)
      |     last = datestr(now,'yyyy');
      | else
      |     last = last(end-3:end);
      | end
      | 
      | if strcmp(first,last)
      |     fprintf('%s -- Copyright %s Nexteer',NxtrConf,first)
      | else
      |     fprintf('%s -- %s%s- %s Nexteer',NxtrConf,char(169),first,last)
      | end
  ElpseTi : Subsystem
  If1 : If  NumInputs=2  IfExpression=u1&u2
  Merge3 : Merge
  RefTi : Subsystem
  Out1 : Outport
  wires:
  Merge3/1 -> Out1/1
  RefTi/1(Out1) -> Merge3/2
  ElpseTi/1(Out1) -> Merge3/1
  If1/2 -> RefTi/Action
  If1/1 -> ElpseTi/Action
  In1/1 -> If1/1
  In2/1 -> If1/2

== system CF009A_GmOvrlStMgr/GmOvrlStMgr/GmOvrlStMgrPer1/HwAgServo ==
  HwAgTrajEna : Inport
  ApaSt : Inport  Port=2
  HwAgTraj : Inport  Port=3
  HwAgTarLimd : Inport  Port=4
  CopyRight2 : Subsystem  Description=|  mask(Copyright Information){none=on}
      | Copyright info block.                                               
      |                                                                     
      | Place copyright information at the top of every subsystem in design.
      mask prompts: none "No parameters"
      mask help: Place copyright information at the top of every subsystem in design.
      mask Display:
      | NxtrConf = 'Nexteer Confidential';
      | 
      | sys = bdroot; %handle for the current model ("system")
      | first = get_param(sys,'Created');
      | if(isempty(first))
      |     first = datestr(now,'yyyy');
      | else
      |     first = first(end-3:end);  %year is last four digits
      | end
      | 
      | last = get_param(sys,'LastModifiedDate');
      | if isempty(last)
      |     last = datestr(now,'yyyy');
      | else
      |     last = last(end-3:end);
      | end
      | 
      | if strcmp(first,last)
      |     fprintf('%s -- Copyright %s Nexteer',NxtrConf,first)
      | else
      |     fprintf('%s -- %s%s- %s Nexteer',NxtrConf,char(169),first,last)
      | end
  If : If  IfExpression=u1
  If Action Subsystem : Subsystem  TreatAsAtomicUnit=on
  If Action Subsystem1 : Subsystem  TreatAsAtomicUnit=on
  Merge : Merge
  Merge1 : Merge
  HwAgServoEna : Outport
  HwAgServoCmd : Outport  Port=2
  wires:
  HwAgTrajEna/1 -> If/1
  If/1 -> If Action Subsystem/Action
  If/2 -> If Action Subsystem1/Action
  HwAgTraj/1 -> If Action Subsystem/2(HwAgTraj)
  ApaSt/1 -> [ApaSt]
  [ApaSt] -> If Action Subsystem/1(ApaSt)
  [ApaSt] -> If Action Subsystem1/1(ApaSt)
  HwAgTarLimd/1 -> If Action Subsystem1/2(HwAgTarLimd)
  If Action Subsystem1/1(HwAgServoCmd) -> Merge/2
  If Action Subsystem/2(HwAgServoCmd) -> Merge/1
  Merge/1 -> HwAgServoCmd/1
  If Action Subsystem/1(HwAgServoEna) -> Merge1/1
  If Action Subsystem1/2(HwAgServoEna) -> Merge1/2
  Merge1/1 -> HwAgServoEna/1

== system CF009A_GmOvrlStMgr/GmOvrlStMgr/GmOvrlStMgrPer1/HwAgTarLimiter ==
  EotCw : Inport
  EotCcw : Inport  Port=2
  HwAgTar : Inport  Port=3
  Add : Sum
  Add1 : Sum  Inputs=-+
  Constant : Constant  RequirementInfo={} %GIDa_d3a7d11a_87b1_4e55_a36f_a3c22d1abccd  Value=GmOvrlStMgrHwAgTarLimr
  CopyRight2 : Subsystem  Description=|  mask(Copyright Information){none=on}
      | Copyright info block.                                               
      |                                                                     
      | Place copyright information at the top of every subsystem in design.
      mask prompts: none "No parameters"
      mask help: Place copyright information at the top of every subsystem in design.
      mask Display:
      | NxtrConf = 'Nexteer Confidential';
      | 
      | sys = bdroot; %handle for the current model ("system")
      | first = get_param(sys,'Created');
      | if(isempty(first))
      |     first = datestr(now,'yyyy');
      | else
      |     first = first(end-3:end);  %year is last four digits
      | end
      | 
      | last = get_param(sys,'LastModifiedDate');
      | if isempty(last)
      |     last = datestr(now,'yyyy');
      | else
      |     last = last(end-3:end);
      | end
      | 
      | if strcmp(first,last)
      |     fprintf('%s -- Copyright %s Nexteer',NxtrConf,first)
      | else
      |     fprintf('%s -- %s%s- %s Nexteer',NxtrConf,char(169),first,last)
      | end
  LimDyn_f32 : NxtrLim/LimDyn_f32
  HwAgTarLimd : Outport
  wires:
  Add/1 -> LimDyn_f32/2
  Add1/1 -> LimDyn_f32/3
  HwAgTar/1 -> LimDyn_f32/1
  LimDyn_f32/1 -> HwAgTarLimd/1
  EotCcw/1 -> Add/1
  Constant/1 -> Add1/1, Add/2
  EotCw/1 -> Add1/2

== system CF009A_GmOvrlStMgr/GmOvrlStMgr/GmOvrlStMgrPer1/HwTqFildIntlChk ==
  In1 : Inport
  Abslt_f32_f32 : NxtrAbslt/Abslt_f32_f32  SFunctionSpec=single y1 = Abslt_f32_f32(single u1)
      settings: AttributesFormatString=%<Name>
  CopyRight2 : Subsystem  Description=|  mask(Copyright Information){none=on}
      | Copyright info block.                                               
      |                                                                     
      | Place copyright information at the top of every subsystem in design.
      mask prompts: none "No parameters"
      mask help: Place copyright information at the top of every subsystem in design.
      mask Display:
      | NxtrConf = 'Nexteer Confidential';
      | 
      | sys = bdroot; %handle for the current model ("system")
      | first = get_param(sys,'Created');
      | first = first(end-3:end);  %year is last four digits
      | 
      | last = get_param(sys,'LastModifiedDate');
      | if isempty(last)
      |     last = datestr(now,'yyyy');
      | else
      |     last = last(end-3:end);
      | end
      | 
      | if strcmp(first,last)
      |     fprintf('%s -- Copyright %s Nexteer',NxtrConf,first)
      | else
      |     fprintf('%s -- %s%s- %s Nexteer',NxtrConf,char(169),first,last)
      | end
  FilLpUpdOutp : Fil/FilLpUpdOutp  StVar=HwTqOscnLpFil
      settings: AttributesFormatString=StVar: %<StVar>
  Interval Test4 : simulink/Logic and Bit Operations/Interval Test  IntervalClosedRight=on  uplimit=GmOvrlStMgrLoaMtgtnHaptcFbTqMax  IntervalClosedLeft=on  lowlimit=GmOvrlStMgrLoaMtgtnHaptcFbTqMin  OutDataTypeStr=boolean
  Out1 : Outport
  wires:
  Interval Test4/1 -> Out1/1
  Abslt_f32_f32/1 -> Interval Test4/1
  FilLpUpdOutp/1 -> Abslt_f32_f32/1
  In1/1 -> FilLpUpdOutp/1

== system CF009A_GmOvrlStMgr/GmOvrlStMgr/GmOvrlStMgrPer1/Inct_IgnCntr_Once ==
  IgnCntrLcl : Inport  RequirementInfo={} %GIDa_31be0032_d248_4158_b577_634f04f9b9d9
  Action Port : ActionPort  ActionType=then
  CopyRight2 : Subsystem  Description=|  mask(Copyright Information){none=on}
      | Copyright info block.                                               
      |                                                                     
      | Place copyright information at the top of every subsystem in design.
      mask prompts: none "No parameters"
      mask help: Place copyright information at the top of every subsystem in design.
      mask Display:
      | NxtrConf = 'Nexteer Confidential';
      | 
      | sys = bdroot; %handle for the current model ("system")
      | first = get_param(sys,'Created');
      | if(isempty(first))
      |     first = datestr(now,'yyyy');
      | else
      |     first = first(end-3:end);  %year is last four digits
      | end
      | 
      | last = get_param(sys,'LastModifiedDate');
      | if isempty(last)
      |     last = datestr(now,'yyyy');
      | else
      |     last = last(end-3:end);
      | end
      | 
      | if strcmp(first,last)
      |     fprintf('%s -- Copyright %s Nexteer',NxtrConf,first)
      | else
      |     fprintf('%s -- %s%s- %s Nexteer',NxtrConf,char(169),first,last)
      | end
  Data Store Read1 : DataStoreRead  DataStoreName=IgnCntrUpd
  If20 : If  IfExpression=~u1  ShowElse=off
  IgnCntr : Subsystem  TreatAsAtomicUnit=on
  wires:
  If20/1 -> IgnCntr/Action
  Data Store Read1/1 -> If20/1
  IgnCntrLcl/1 -> IgnCntr/1(IgnCntrLcl)
